simulink model "EKF"  (R2019a)
settings: Solver=FixedStepAuto  StartTime=0.0  StopTime=10.0  RelTol=1e-3
InitFcn:
  | EKF_init
settings Model: Creator=somli  LastModifiedBy=den

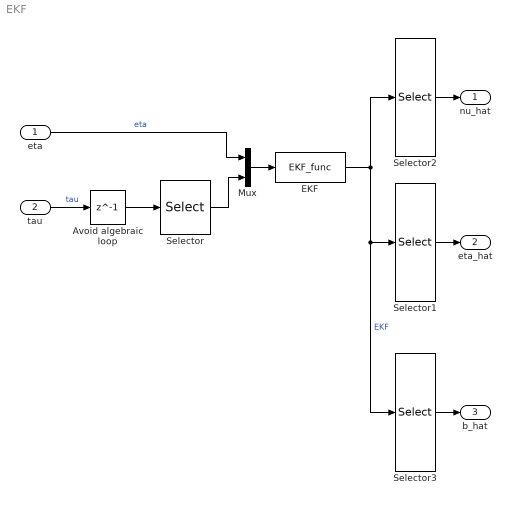
== system EKF ==
  eta : Inport  PortDimensions=3  SampleTime=0.1
  tau : Inport  Port=2  PortDimensions=6  SampleTime=0.1
  Avoid algebraic loop : Delay  DelayLength=1
  EKF : MATLABFcn  MATLABFcn=EKF_func  Output1D=off
  Mux : Mux  Inputs=2
  Selector : Selector  InputPortWidth=6  IndexOptions=Index vector (dialog)  Indices=[1 2 6]  OutputSizes=1
  Selector1 : Selector  InputPortWidth=15  IndexOptions=Index vector (dialog)  Indices=[7:9]  OutputSizes=1
  Selector2 : Selector  InputPortWidth=15  IndexOptions=Index vector (dialog)  Indices=[13:15]  OutputSizes=1
  Selector3 : Selector  InputPortWidth=15  IndexOptions=Index vector (dialog)  Indices=[10:12]  OutputSizes=1
  nu_hat : Outport  PortDimensions=3  SampleTime=0.1
  eta_hat : Outport  Port=2  PortDimensions=3  SampleTime=0.1
  b_hat : Outport  Port=3  PortDimensions=3  SampleTime=0.1
  wires:
  Mux/1 -> EKF/1
  eta/1 -> Mux/1  "eta"
  tau/1 -> Avoid algebraic loop/1  "tau"
  Selector/1 -> Mux/2
  Selector2/1 -> nu_hat/1
  Selector1/1 -> eta_hat/1
  Avoid algebraic loop/1 -> Selector/1
  Selector3/1 -> b_hat/1
  EKF/1 -> Selector3/1, Selector1/1, Selector2/1  "EKF"
